simulink model "fadianjimoxing"  (R2014a)
settings: Solver=ode45  StartTime=0.0  StopTime=10.0  RelTol=1e-3
settings Model: Creator=hsinwang  LastModifiedBy=hsinwang

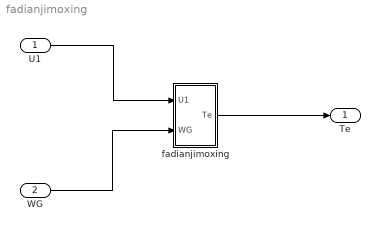
== system fadianjimoxing ==
  U1 : Inport
  WG : Inport  Port=2
  "fadianjimoxing " : Subsystem
  Te : Outport
  wires:
  U1/1 -> "fadianjimoxing "/1(U1)
  WG/1 -> "fadianjimoxing "/2(WG)
  "fadianjimoxing "/1(Te) -> Te/1

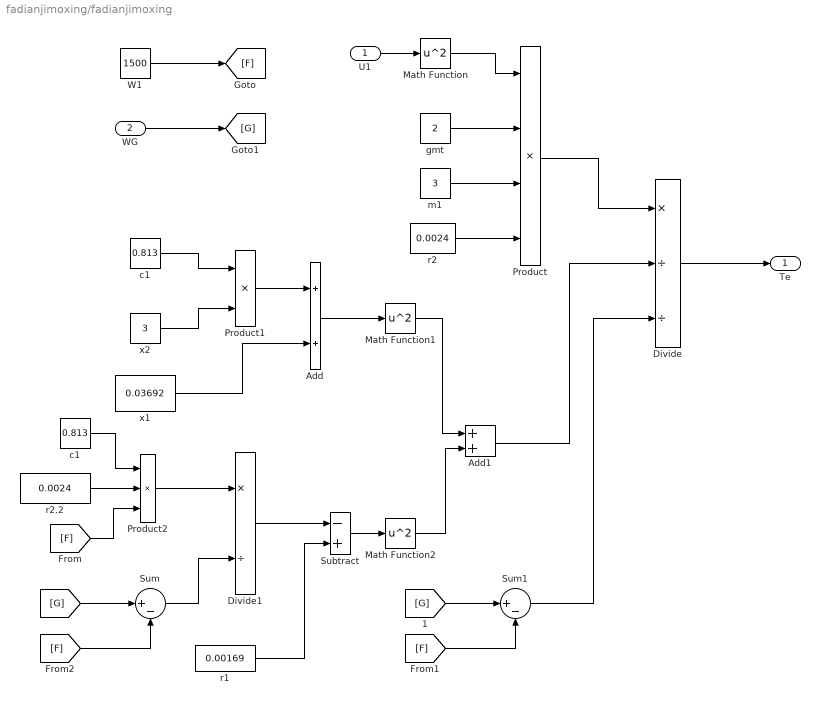
== system fadianjimoxing/fadianjimoxing  ==
  U1 : Inport
  WG : Inport  Port=2
  Add : Sum
  Add1 : Sum
  Divide : Product  Inputs=*//
  Divide1 : Product  Inputs=*/
  Math Function : Math  Operator=square  SaturateOnIntegerOverflow=on
  Math Function1 : Math  Operator=square  SaturateOnIntegerOverflow=on
  Math Function2 : Math  Operator=square  SaturateOnIntegerOverflow=on
  Product : Product  Inputs=4
  Product1 : Product
  Product2 : Product  Inputs=3
  Subtract : Sum  Inputs=-+
  Sum : Sum  Inputs=|+-
  Sum1 : Sum  Inputs=|+-
  W1 : Constant  Value=1500
  c1 : Constant  Value=0.813
  "c1 " : Constant  Value=0.813
  gmt : Constant  Value=2
  m1 : Constant  Value=3
  r1 : Constant  Value=0.00169
  r2 : Constant  Value=0.0024
  r2.2 : Constant  Value=0.0024
  "x1 " : Constant  Value=0.03692
  x2 : Constant  Value=3
  Te : Outport
  wires:
  r2/1 -> Product/4
  Math Function/1 -> Product/1
  m1/1 -> Product/3
  "x1 "/1 -> Add/2
  gmt/1 -> Product/2
  Math Function1/1 -> Add1/1
  Math Function2/1 -> Add1/2
  [F] -> Sum1/2
  [G] -> Sum1/1
  Sum1/1 -> Divide/3
  c1/1 -> Product2/1
  [F] -> Product2/3
  [G] -> Sum/1
  Divide1/1 -> Subtract/1
  [F] -> Sum/2
  r1/1 -> Subtract/2
  r2.2/1 -> Product2/2
  Product2/1 -> Divide1/1
  Add1/1 -> Divide/2
  Subtract/1 -> Math Function2/1
  W1/1 -> [F]
  Product/1 -> Divide/1
  "c1 "/1 -> Product1/1
  Divide/1 -> Te/1
  x2/1 -> Product1/2
  WG/1 -> [G]
  Add/1 -> Math Function1/1
  U1/1 -> Math Function/1
  Sum/1 -> Divide1/2
  Product1/1 -> Add/1
